simulink model "proyectoscada"  (R2016b)
settings: Solver=VariableStepAuto  StartTime=0.0  StopTime=inf  RelTol=1e-3
undefined symbols (not defined in the file): D1, Delta
libraries: powerlib x32, powerlib_meascontrol x17, sps_avr x2
settings Model: Creator=Chabla  LastModifiedBy=Chabla

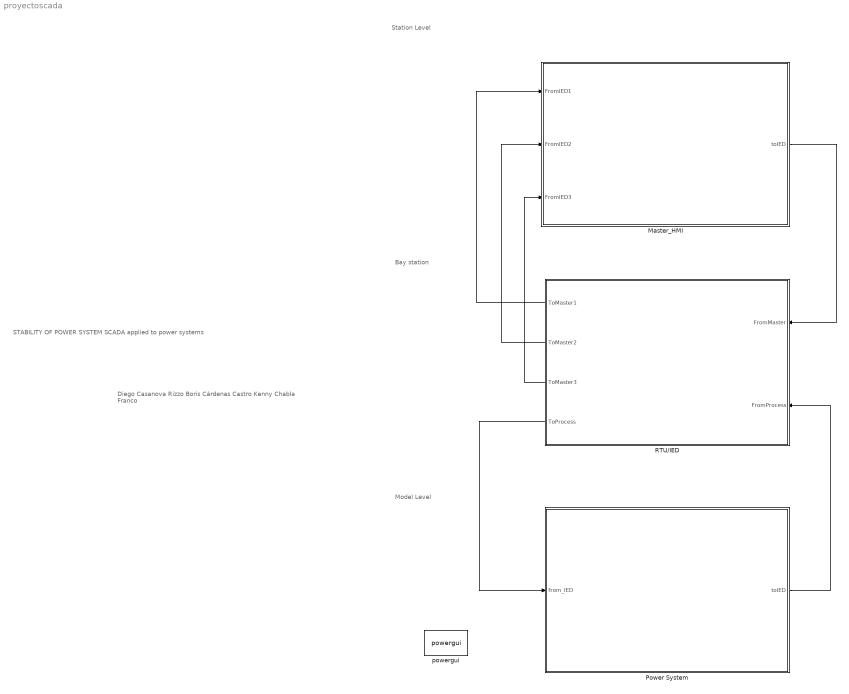
== system proyectoscada ==
  note: Station Level
  note: Bay station
  note: Model Level
  note: STABILITY OF POWER SYSTEM
      | SCADA applied to power systems
  note: Diego Casanova Rizzo
      | Boris Cárdenas Castro
      | Kenny Chabla Franco
  Master_HMI : Subsystem
  Power System : Subsystem
  RTU/IED : Subsystem
  powergui : powerlib/powergui  Priority=1  SimulationMode=Discrete  SolverType=Tustin/Backward Euler (TBE)  SampleTime=50e-6  frequency=60  SPID=off  DisableSnubberDevices=off  DisableRonSwitches=off  DisableVfSwitches=off  SwTol=0  DisplayEquations=off  Interpol=off  ExternalGateDelay=off  methode=off  Ts=10  FunctionMessages=off  echomessages=off  HookPort=off  EnableUseOfTLC=off  x0status=blocks  frequencyindice=60  Pbase=100e6  ErrMax=1e-4  Iterations=50  UnitsV=kV  UnitsW=MW  buscounter=0  RestoreLinks=warning  ResistiveCurrentMeasurement=off  Frange=[0:2:500]  Ylog=off  Xlog=on  ShowGrid=off  save=off  variable=ZData  structure=0  ZoomFFT=off  StartTime=0.0  cycles=1  DisplayStyle=1  fundamental=60  FreqAxis=off  MaxFrequency=1000  frequencyindicesteady=1  RmsSteady=1  display=off
  wires:
  RTU/IED/4(ToProcess) -> Power System/1(from_IED)
  Power System/1(toIED) -> RTU/IED/2(FromProcess)
  RTU/IED/1(ToMaster1) -> Master_HMI/1(FromIED1)
  Master_HMI/1(toIED) -> RTU/IED/1(FromMaster)
  RTU/IED/2(ToMaster2) -> Master_HMI/2(FromIED2)
  RTU/IED/3(ToMaster3) -> Master_HMI/3(FromIED3)

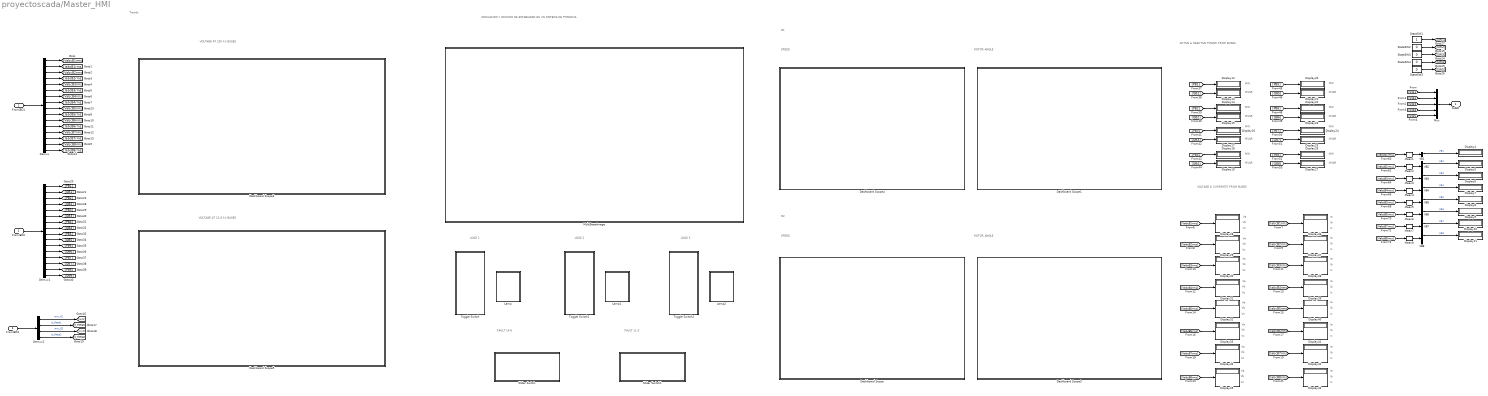
== system proyectoscada/Master_HMI ==
  note: SIMULACIÓN Y ESTUDIO DE ESTABILIDAD
      | EN UN SISTEMA DE POTENCIA
  note: LOAD 1
  note: LOAD 2
  note: LOAD 3
  note: FAULT L4-6
  note: FAULT L1-3
  note: G1
  note: SPEED
  note: ROTOR ANGLE
  note: G2
  note: SPEED
  note: ROTOR ANGLE
  note: ACTIVE & REACTIVE POWER
      | FROM BUSES
  note: VOLTAGE & CURRENTS
      | FROM BUSES
  note: VOLTAGE AT 230 kV BUSES
  note: VOLTAGE AT 13.8 kV BUSES
  note: Trends
  note: MW
  note: MW
  note: MW
  note: MW
  note: MW
  note: MW
  note: MVAR
  note: MVAR
  note: MVAR
  note: MVAR
  note: MVAR
  note: MVAR
  note: MW
  note: MW
  note: MVAR
  note: MVAR
  note: Va
  note: Vb
  note: Vc
  note: Va
  note: Vb
  note: Vc
  note: Va
  note: Vb
  note: Vc
  note: Va
  note: Vb
  note: Vc
  note: Va
  note: Vb
  note: Vc
  note: Va
  note: Vb
  note: Vc
  note: Va
  note: Vb
  note: Vc
  note: Va
  note: Vb
  note: Vc
  note: Ia
  note: Ib
  note: Ic
  note: Ia
  note: Ib
  note: Ic
  note: Ia
  note: Ib
  note: Ic
  note: Ia
  note: Ib
  note: Ic
  note: Ia
  note: Ib
  note: Ic
  note: Ia
  note: Ib
  note: Ic
  note: Ia
  note: Ib
  note: Ic
  note: Ia
  note: Ib
  note: Ic
  FromIED1 : Inport
  FromIED2 : Inport  Port=2
  FromIED3 : Inport  Port=3
  Dashboard Scope : Subsystem  DialogController=hmiCreateDDGDialog  IsWebBlock=on  mask(MWDashboardBlock){webBlockId=cafc33a1-a38a-4801-83e7-bfcad2fb4042, webBlockType=sdiscope, ShowInitialText=on, HMISrcModelName=proyectoscada_primerparcial}
      mask prompts: webBlockId "WebBlock Id"; webBlockType "WebBlock Type"; HMISrcModelName "Source Model"
      mask help: SimulinkHMI:dialogs:HMIScopeDialogDesc
      mask Help: helpview([docroot '/mapfiles/simulink.map'], 'hmi_scope')
      mask Display:
      | if strcmp(get_param(bdroot(gcb),'BlockDiagramType'), 'library')
      |     image([(matlabroot) '/toolbox/simulink/hmi/icons/DashboardScope.png']);
      | end
  Dashboard Scope1 : Subsystem  DialogController=hmiCreateDDGDialog  IsWebBlock=on  mask(MWDashboardBlock){webBlockId=1f27aae5-dc6e-47fc-b79d-12c84d4126a5, webBlockType=sdiscope, ShowInitialText=on, HMISrcModelName=proyectoscada_primerparcial}
      mask prompts: webBlockId "WebBlock Id"; webBlockType "WebBlock Type"; HMISrcModelName "Source Model"
      mask help: SimulinkHMI:dialogs:HMIScopeDialogDesc
      mask Help: helpview([docroot '/mapfiles/simulink.map'], 'hmi_scope')
      mask Display:
      | if strcmp(get_param(bdroot(gcb),'BlockDiagramType'), 'library')
      |     image([(matlabroot) '/toolbox/simulink/hmi/icons/DashboardScope.png']);
      | end
  Dashboard Scope2 : Subsystem  DialogController=hmiCreateDDGDialog  IsWebBlock=on  mask(MWDashboardBlock){webBlockId=bb99fa04-7dbe-4198-be6d-771c31951309, webBlockType=sdiscope, ShowInitialText=off, HMISrcModelName=proyectoscada_primerparcial}
      mask prompts: webBlockId "WebBlock Id"; webBlockType "WebBlock Type"; HMISrcModelName "Source Model"
      mask help: SimulinkHMI:dialogs:HMIScopeDialogDesc
      mask Help: helpview([docroot '/mapfiles/simulink.map'], 'hmi_scope')
      mask Display:
      | if strcmp(get_param(bdroot(gcb),'BlockDiagramType'), 'library')
      |     image([(matlabroot) '/toolbox/simulink/hmi/icons/DashboardScope.png']);
      | end
  Dashboard Scope3 : Subsystem  DialogController=hmiCreateDDGDialog  IsWebBlock=on  mask(MWDashboardBlock){webBlockId=8463cc78-291a-42f6-a448-124f53d8cf61, webBlockType=sdiscope, ShowInitialText=on, HMISrcModelName=proyectoscada_primerparcial}
      mask prompts: webBlockId "WebBlock Id"; webBlockType "WebBlock Type"; HMISrcModelName "Source Model"
      mask help: SimulinkHMI:dialogs:HMIScopeDialogDesc
      mask Help: helpview([docroot '/mapfiles/simulink.map'], 'hmi_scope')
      mask Display:
      | if strcmp(get_param(bdroot(gcb),'BlockDiagramType'), 'library')
      |     image([(matlabroot) '/toolbox/simulink/hmi/icons/DashboardScope.png']);
      | end
  Dashboard Scope4 : Subsystem  DialogController=hmiCreateDDGDialog  IsWebBlock=on  mask(MWDashboardBlock){webBlockId=24e836a3-7620-49fe-a566-1de62ba9f4e1, webBlockType=sdiscope, ShowInitialText=on, HMISrcModelName=proyectoscada_primerparcial}
      mask prompts: webBlockId "WebBlock Id"; webBlockType "WebBlock Type"; HMISrcModelName "Source Model"
      mask help: SimulinkHMI:dialogs:HMIScopeDialogDesc
      mask Help: helpview([docroot '/mapfiles/simulink.map'], 'hmi_scope')
      mask Display:
      | if strcmp(get_param(bdroot(gcb),'BlockDiagramType'), 'library')
      |     image([(matlabroot) '/toolbox/simulink/hmi/icons/DashboardScope.png']);
      | end
  Dashboard Scope5 : Subsystem  DialogController=hmiCreateDDGDialog  IsWebBlock=on  mask(MWDashboardBlock){webBlockId=cad27841-eb8e-42d3-b755-ee1d88cca136, webBlockType=sdiscope, ShowInitialText=off, HMISrcModelName=proyectoscada_primerparcial}
      mask prompts: webBlockId "WebBlock Id"; webBlockType "WebBlock Type"; HMISrcModelName "Source Model"
      mask help: SimulinkHMI:dialogs:HMIScopeDialogDesc
      mask Help: helpview([docroot '/mapfiles/simulink.map'], 'hmi_scope')
      mask Display:
      | if strcmp(get_param(bdroot(gcb),'BlockDiagramType'), 'library')
      |     image([(matlabroot) '/toolbox/simulink/hmi/icons/DashboardScope.png']);
      | end
  Demux : Demux  Outputs=16
  Demux1 : Demux  Outputs=16
  Demux2 : Demux
  Display{4..43} (40 alike) : Display
      settings: Format=bank  Decimation=2
  Lamp : Subsystem  DialogController=hmiCreateDDGDialog  IsWebBlock=on  mask(MWDashboardBlock){webBlockId=6d0128fc-3d43-4d5e-b84a-a99f5afbf392, webBlockType=lamp, ShowInLibBrowser=on, ShowInitialText=on, HMISrcModelName=proyectoscada_primerparcial}
      mask prompts: webBlockType "WebBlock Type"; HMISrcModelName "Source Model"
      mask help: SimulinkHMI:dialogs:LampDialogDesc
      mask Help: helpview([docroot '/mapfiles/simulink.map'], 'hmi_lamp')
      mask Display:
      | if strcmp(get_param(bdroot(gcb),'BlockDiagramType'), 'library')
      |     image([(matlabroot) '/toolbox/simulink/hmi/icons/Lamp.png']);
      | end
  Lamp1 : Subsystem  DialogController=hmiCreateDDGDialog  IsWebBlock=on  mask(MWDashboardBlock){webBlockId=c150fd86-0204-4bcb-8bb8-b9940914ece7, webBlockType=lamp, ShowInLibBrowser=on, ShowInitialText=on, HMISrcModelName=proyectoscada_primerparcial}
      mask prompts: webBlockType "WebBlock Type"; HMISrcModelName "Source Model"
      mask help: SimulinkHMI:dialogs:LampDialogDesc
      mask Help: helpview([docroot '/mapfiles/simulink.map'], 'hmi_lamp')
      mask Display:
      | if strcmp(get_param(bdroot(gcb),'BlockDiagramType'), 'library')
      |     image([(matlabroot) '/toolbox/simulink/hmi/icons/Lamp.png']);
      | end
  Lamp2 : Subsystem  DialogController=hmiCreateDDGDialog  IsWebBlock=on  mask(MWDashboardBlock){webBlockId=436e8146-0c8e-45d0-95ec-43b164432763, webBlockType=lamp, ShowInLibBrowser=on, ShowInitialText=on, HMISrcModelName=proyectoscada_primerparcial}
      mask prompts: webBlockType "WebBlock Type"; HMISrcModelName "Source Model"
      mask help: SimulinkHMI:dialogs:LampDialogDesc
      mask Help: helpview([docroot '/mapfiles/simulink.map'], 'hmi_lamp')
      mask Display:
      | if strcmp(get_param(bdroot(gcb),'BlockDiagramType'), 'library')
      |     image([(matlabroot) '/toolbox/simulink/hmi/icons/Lamp.png']);
      | end
  Mean{1..8} (8 alike) : powerlib_meascontrol/Measurements/Mean  Freq=60  Vinit=0  Ts=0
  MultiStateImage : Subsystem  DialogController=hmiCreateDDGDialog  IsWebBlock=on  mask(MWDashboardBlock){webBlockId=108d4e63-1026-47ee-835d-08ebfdb5bc59, webBlockType=multistateimage, ShowInLibBrowser=on, ShowInitialText=on, HMISrcModelName=proyectoscada_primerparcial}
      mask prompts: webBlockType "WebBlock Type"; HMISrcModelName "Source Model"
      mask help: SimulinkHMI:dialogs:MultiStateImageDialogDesc
      mask Help: helpview([docroot '/mapfiles/simulink.map'], 'hmi_multistateimage')
      mask Display:
      | if strcmp(get_param(bdroot(gcb),'BlockDiagramType'), 'library')
      |     image([(matlabroot) '/toolbox/simulink/hmi/icons/MultiStateImage.png']);
      | end
  Mux : Mux  Inputs=5
  Slider Switch : Subsystem  DialogController=hmiCreateDDGDialog  IsWebBlock=on  mask(MWDashboardBlock){webBlockId=03720d25-6366-4281-ad77-0615db862108, webBlockType=sliderswitch, ShowInLibBrowser=on, ShowInitialText=on, HMISrcModelName=proyectoscada_primerparcial}
      mask prompts: webBlockId "WebBlock Id"; webBlockType "WebBlock Type"; HMISrcModelName "Source Model"
      mask help: SimulinkHMI:dialogs:SwitchDialogDesc
      mask Help: helpview([docroot '/mapfiles/simulink.map'], 'hmi_slider_switch')
      mask Display:
      | if strcmp(get_param(bdroot(gcb),'BlockDiagramType'), 'library')
      |     image([(matlabroot) '/toolbox/simulink/hmi/icons/SliderSwitch.png']);
      | end
  Slider Switch1 : Subsystem  DialogController=hmiCreateDDGDialog  IsWebBlock=on  mask(MWDashboardBlock){webBlockId=6740b061-e7b1-413b-8a03-3a4303ef55f0, webBlockType=sliderswitch, ShowInLibBrowser=on, ShowInitialText=on, HMISrcModelName=proyectoscada_primerparcial}
      mask prompts: webBlockId "WebBlock Id"; webBlockType "WebBlock Type"; HMISrcModelName "Source Model"
      mask help: SimulinkHMI:dialogs:SwitchDialogDesc
      mask Help: helpview([docroot '/mapfiles/simulink.map'], 'hmi_slider_switch')
      mask Display:
      | if strcmp(get_param(bdroot(gcb),'BlockDiagramType'), 'library')
      |     image([(matlabroot) '/toolbox/simulink/hmi/icons/SliderSwitch.png']);
      | end
  StateSW1 : Constant
  StateSW{2..5} (4 alike) : Constant  Value=0
  Toggle Switch : Subsystem  DialogController=hmiCreateDDGDialog  IsWebBlock=on  mask(MWDashboardBlock){webBlockId=0404eeae-805f-465c-bc8a-4052b3d66771, webBlockType=toggleswitch, ShowInLibBrowser=on, ShowInitialText=on, HMISrcModelName=proyectoscada_primerparcial}
      mask prompts: webBlockId "WebBlock Id"; webBlockType "WebBlock Type"; HMISrcModelName "Source Model"
      mask help: SimulinkHMI:dialogs:SwitchDialogDesc
      mask Help: helpview([docroot '/mapfiles/simulink.map'], 'hmi_toggle_switch')
      mask Display:
      | if strcmp(get_param(bdroot(gcb),'BlockDiagramType'), 'library')
      |     image([(matlabroot) '/toolbox/simulink/hmi/icons/ToggleSwitch.png']);
      | end
  Toggle Switch1 : Subsystem  DialogController=hmiCreateDDGDialog  IsWebBlock=on  mask(MWDashboardBlock){webBlockId=4eb36801-e82a-44a6-9453-5649fb68f4bc, webBlockType=toggleswitch, ShowInLibBrowser=on, ShowInitialText=on, HMISrcModelName=proyectoscada_primerparcial}
      mask prompts: webBlockId "WebBlock Id"; webBlockType "WebBlock Type"; HMISrcModelName "Source Model"
      mask help: SimulinkHMI:dialogs:SwitchDialogDesc
      mask Help: helpview([docroot '/mapfiles/simulink.map'], 'hmi_toggle_switch')
      mask Display:
      | if strcmp(get_param(bdroot(gcb),'BlockDiagramType'), 'library')
      |     image([(matlabroot) '/toolbox/simulink/hmi/icons/ToggleSwitch.png']);
      | end
  Toggle Switch2 : Subsystem  DialogController=hmiCreateDDGDialog  IsWebBlock=on  mask(MWDashboardBlock){webBlockId=05c27441-99b6-4173-8686-6e6faba039f7, webBlockType=toggleswitch, ShowInLibBrowser=on, ShowInitialText=on, HMISrcModelName=proyectoscada_primerparcial}
      mask prompts: webBlockId "WebBlock Id"; webBlockType "WebBlock Type"; HMISrcModelName "Source Model"
      mask help: SimulinkHMI:dialogs:SwitchDialogDesc
      mask Help: helpview([docroot '/mapfiles/simulink.map'], 'hmi_toggle_switch')
      mask Display:
      | if strcmp(get_param(bdroot(gcb),'BlockDiagramType'), 'library')
      |     image([(matlabroot) '/toolbox/simulink/hmi/icons/ToggleSwitch.png']);
      | end
  VB{1..8} (8 alike) : Demux  Outputs=3
  toIED : Outport
  wires:
  FromIED1/1 -> Demux/1
  Demux/1 -> [VabcB1rms]
  Demux/2 -> [IabcB1rms]
  Demux/3 -> [VabcB2rms]
  Demux/4 -> [IabcB2rms]
  Demux/5 -> [VabcB3rms]
  Demux/6 -> [IabcB3rms]
  Demux/7 -> [VabcB4rms]
  Demux/8 -> [IabcB4rms]
  Demux/9 -> [VabcB5rms]
  Demux/10 -> [IabcB5rms]
  Demux/11 -> [VabcB6rms]
  Demux/12 -> [IabcB6rms]
  Demux/13 -> [VabcB7rms]
  Demux/14 -> [IabcB7rms]
  Demux/15 -> [VabcB8rms]
  Demux/16 -> [IabcB8rms]
  Demux1/1 -> [PB1]
  Demux1/2 -> [QB1]
  Demux1/3 -> [PB2]
  Demux1/4 -> [QB2]
  Demux1/5 -> [PB3]
  Demux1/6 -> [QB3]
  Demux1/7 -> [PB4]
  Demux1/8 -> [QB4]
  Demux1/9 -> [PB5]
  Demux1/10 -> [QB5]
  Demux1/11 -> [PB6]
  Demux1/12 -> [QB6]
  Demux1/13 -> [PB7]
  Demux1/14 -> [QB7]
  Demux1/15 -> [PB8]
  Demux1/16 -> [QB8]
  FromIED2/1 -> Demux1/1
  Demux2/2 -> [d_theta1]  "d_theta1"
  Demux2/4 -> [d_theta2]  "d_theta2"
  Demux2/1 -> [wm]  "wm_G1"
  Demux2/3 -> [wm2]  "wm_G2"
  FromIED3/1 -> Demux2/1
  Mux/1 -> toIED/1
  [SW1] -> Mux/1
  [SW2] -> Mux/2
  [SW3] -> Mux/3
  [SW4] -> Mux/4
  [SW5] -> Mux/5
  StateSW1/1 -> [SW1]
  StateSW2/1 -> [SW2]
  StateSW3/1 -> [SW3]
  StateSW4/1 -> [SW4]
  StateSW5/1 -> [SW5]
  [VabcB1rms] -> Mean1/1
  Mean1/1 -> VB1/1
  Mean2/1 -> VB2/1
  Mean3/1 -> VB3/1
  Mean4/1 -> VB4/1
  Mean5/1 -> VB5/1
  Mean6/1 -> VB6/1
  Mean7/1 -> VB7/1
  Mean8/1 -> VB8/1
  [VabcB2rms] -> Mean2/1
  [VabcB3rms] -> Mean3/1
  [VabcB4rms] -> Mean4/1
  [VabcB8rms] -> Mean8/1
  [VabcB7rms] -> Mean7/1
  [VabcB6rms] -> Mean6/1
  [VabcB5rms] -> Mean5/1
  VB1/1 -> Display4/1  "VB1"
  VB2/1 -> Display5/1  "VB2"
  VB3/1 -> Display6/1  "VB3"
  VB4/1 -> Display7/1  "VB4"
  VB5/1 -> Display8/1  "VB5"
  VB6/1 -> Display9/1  "VB6"
  VB7/1 -> Display10/1  "VB7"
  VB8/1 -> Display11/1  "VB8"
  [QB1] -> Display13/1
  [PB2] -> Display14/1
  [QB2] -> Display15/1
  [PB3] -> Display16/1
  [QB3] -> Display17/1
  [PB4] -> Display18/1
  [QB4] -> Display19/1
  [PB5] -> Display20/1
  [QB5] -> Display21/1
  [PB6] -> Display22/1
  [QB6] -> Display23/1
  [PB7] -> Display24/1
  [QB7] -> Display25/1
  [PB8] -> Display26/1
  [QB8] -> Display27/1
  [VabcB1rms] -> Display28/1
  [VabcB2rms] -> Display29/1
  [VabcB3rms] -> Display30/1
  [VabcB4rms] -> Display31/1
  [VabcB5rms] -> Display32/1
  [VabcB6rms] -> Display33/1
  [VabcB7rms] -> Display34/1
  [VabcB8rms] -> Display35/1
  [IabcB1rms] -> Display36/1
  [IabcB2rms] -> Display37/1
  [IabcB3rms] -> Display38/1
  [IabcB4rms] -> Display39/1
  [IabcB5rms] -> Display40/1
  [IabcB6rms] -> Display41/1
  [IabcB7rms] -> Display42/1
  [IabcB8rms] -> Display43/1
  [PB1] -> Display12/1

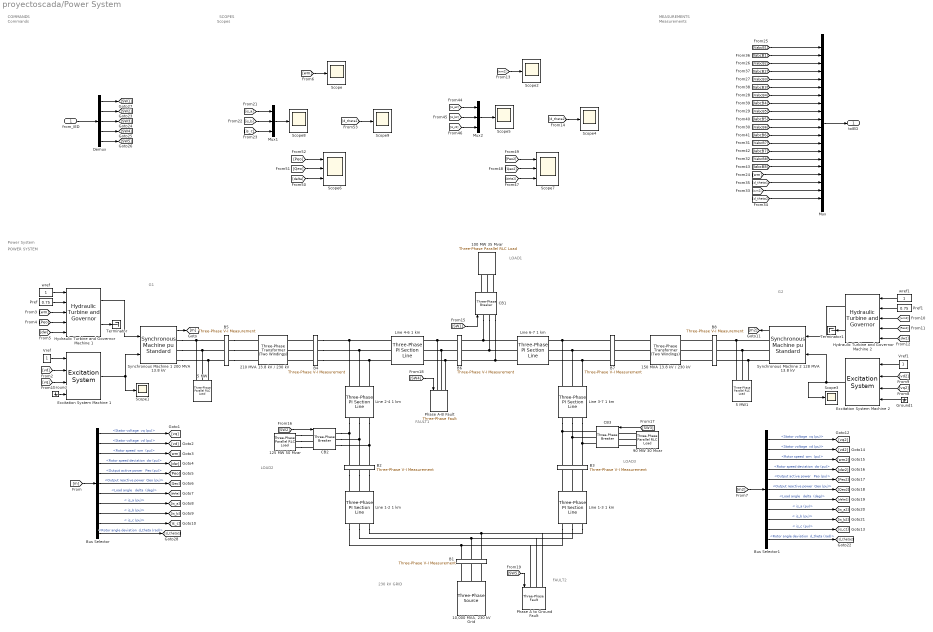
== system proyectoscada/Power System ==
  note: G1
  note: Scopes
  note: Measurements
  note: Power System
  note: Commands
  note: G2
  note: 230 kV
      | GRID
  note: LOAD1
  note: LOAD2
  note: LOAD3
  note: FAULT1
  note: FAULT2
  note: COMMANDS
  note: SCOPES
  note: MEASUREMENTS
  note: POWER SYSTEM
  from_IED : Inport
  "10,000 MVA, 230 kV Grid" : powerlib/Electrical Sources/Three-Phase Source  InternalConnection=Yg  VoltagePhases=off  Voltage=(230000)*1.00006  PhaseAngle=-0.77547  Voltage_phases=[25e3 25e3 25e3]/sqrt(3)  PhaseAngles_phases=[0 -120 +120]  Frequency=60  NonIdealSource=on  SpecifyImpedance=on  Resistance=0.529  Inductance=0.0140  ShortCircuitLevel=10000e6  BaseVoltage=230e3  XRratio=10  BusType=swing  Pref=0  Qref=0  Prefabc=[10e3, 10e3, 10e3]  Qrefabc=[0, 0, 0]  Qmin=-Inf  Qmax=Inf
  100 MW 35 Mvar : powerlib/Elements/Three-Phase Parallel RLC Load  LConnTagsString=A|B|C  Configuration=Y (grounded)  NominalVoltage=230e3  Vabc=[1e3 1e3 1e3]  Vabcp=[1e3 1e3 1e3]  NominalFrequency=60  UnbalancedPower=off  ActivePower=100000000  InductivePower=35000000  CapacitivePower=0  Pabc=[10e3 9e3 11e3]  QLabc=[100 90 110]  QCabc=[100 90 110]  Pabcp=[10e3 9e3 11e3]  QLabcp=[100 90 110]  QCabcp=[100 90 110]  Measurements=None  LoadType=constant Z
  125 MW 50 Mvar : powerlib/Elements/Three-Phase Parallel RLC Load  LConnTagsString=A|B|C  Configuration=Y (grounded)  NominalVoltage=230e3  Vabc=[1e3 1e3 1e3]  Vabcp=[1e3 1e3 1e3]  NominalFrequency=60  UnbalancedPower=off  ActivePower=125000000  InductivePower=50000000  CapacitivePower=0  Pabc=[10e3 9e3 11e3]  QLabc=[100 90 110]  QCabc=[100 90 110]  Pabcp=[10e3 9e3 11e3]  QLabcp=[100 90 110]  QCabcp=[100 90 110]  Measurements=None  LoadType=constant Z
  150 MVA 13.8 kV / 230 kV : powerlib/Elements/Three-Phase Transformer (Two Windings)  Winding1Connection=Delta (D1)  Winding2Connection=Yg  CoreType=Three single-phase transformers  SetSaturation=off  Hysteresis=off  DataFile='hysteresis'  SetInitialFlux=off  Measurements=None  UNITS=pu  NominalPower=[ 150e6 60 ]  Winding1="[ 13.8e3 0.0027  0.08]"  Winding2=[ 230e3 0.0027 0.08]  Rm=500  Lm=500  L0=0.5  Saturation="[ 0,0  ;  0.005,1.2  ;  1.0,1.4 ]"  InitialFluxes=[ 0.8 , -0.8 , 0.7 ]  MoreParameters=off  BreakLoop=off  DataType=off  TransfoNumber=0
  210 MVA 13.8 kV / 230 kV : powerlib/Elements/Three-Phase Transformer (Two Windings)  Winding1Connection=Delta (D1)  Winding2Connection=Yg  CoreType=Three single-phase transformers  SetSaturation=off  Hysteresis=off  DataFile='hysteresis'  SetInitialFlux=off  Measurements=None  UNITS=pu  NominalPower=[ 210e6 60 ]  Winding1="[ 13.8e3 0.0027  0.08]"  Winding2=[ 230e3 0.0027 0.08]  Rm=500  Lm=500  L0=0.5  Saturation="[ 0,0  ;  0.005,1.2  ;  1.0,1.4 ]"  InitialFluxes=[ 0.8 , -0.8 , 0.7 ]  MoreParameters=off  BreakLoop=off  DataType=off  TransfoNumber=0
  5 MW : powerlib/Elements/Three-Phase Parallel RLC Load  LConnTagsString=A|B|C  Configuration=Y (grounded)  NominalVoltage=13.8e3  Vabc=[1e3 1e3 1e3]  Vabcp=[1e3 1e3 1e3]  NominalFrequency=60  UnbalancedPower=off  ActivePower=125000000  InductivePower=0  CapacitivePower=0  Pabc=[10e3 9e3 11e3]  QLabc=[100 90 110]  QCabc=[100 90 110]  Pabcp=[10e3 9e3 11e3]  QLabcp=[100 90 110]  QCabcp=[100 90 110]  Measurements=None  LoadType=constant Z
  5 MW1 : powerlib/Elements/Three-Phase Parallel RLC Load  LConnTagsString=A|B|C  Configuration=Y (grounded)  NominalVoltage=13.8e3  Vabc=[1e3 1e3 1e3]  Vabcp=[1e3 1e3 1e3]  NominalFrequency=60  UnbalancedPower=off  ActivePower=125000000  InductivePower=0  CapacitivePower=0  Pabc=[10e3 9e3 11e3]  QLabc=[100 90 110]  QCabc=[100 90 110]  Pabcp=[10e3 9e3 11e3]  QLabcp=[100 90 110]  QCabcp=[100 90 110]  Measurements=None  LoadType=constant Z
  90 MW 30 Mvar : powerlib/Elements/Three-Phase Parallel RLC Load  LConnTagsString=A|B|C  Configuration=Y (grounded)  NominalVoltage=230e3  Vabc=[1e3 1e3 1e3]  Vabcp=[1e3 1e3 1e3]  NominalFrequency=60  UnbalancedPower=off  ActivePower=90000000  InductivePower=30000000  CapacitivePower=0  Pabc=[10e3 9e3 11e3]  QLabc=[100 90 110]  QCabc=[100 90 110]  Pabcp=[10e3 9e3 11e3]  QLabcp=[100 90 110]  QCabcp=[100 90 110]  Measurements=None  LoadType=constant Z
  B1 : powerlib/Measurements/Three-Phase V-I Measurement  VoltageMeasurement=phase-to-phase  SetLabelV=on  LabelV=VabcB1  Vpu=off  VpuLL=off  CurrentMeasurement=yes  SetLabelI=on  LabelI=IabcB1  Ipu=off  Pbase=100e6  Vbase=500e3  OutputType=Complex  PhasorSimulation=off  PSBequivalent=0
  B2 : powerlib/Measurements/Three-Phase V-I Measurement  VoltageMeasurement=phase-to-phase  SetLabelV=on  LabelV=VabcB2  Vpu=off  VpuLL=off  CurrentMeasurement=yes  SetLabelI=on  LabelI=IabcB2  Ipu=off  Pbase=100e6  Vbase=500e3  OutputType=Complex  PhasorSimulation=off  PSBequivalent=0
  B3 : powerlib/Measurements/Three-Phase V-I Measurement  VoltageMeasurement=phase-to-phase  SetLabelV=on  LabelV=VabcB3  Vpu=off  VpuLL=off  CurrentMeasurement=yes  SetLabelI=on  LabelI=IabcB3  Ipu=off  Pbase=100e6  Vbase=500e3  OutputType=Complex  PhasorSimulation=off  PSBequivalent=0
  B4 : powerlib/Measurements/Three-Phase V-I Measurement  VoltageMeasurement=phase-to-phase  SetLabelV=on  LabelV=VabcB4  Vpu=off  VpuLL=off  CurrentMeasurement=yes  SetLabelI=on  LabelI=IabcB4  Ipu=off  Pbase=100e6  Vbase=500e3  OutputType=Complex  PhasorSimulation=off  PSBequivalent=0
  B5 : powerlib/Measurements/Three-Phase V-I Measurement  VoltageMeasurement=phase-to-phase  SetLabelV=on  LabelV=VabcB5  Vpu=off  VpuLL=off  CurrentMeasurement=yes  SetLabelI=on  LabelI=IabcB5  Ipu=off  Pbase=100e6  Vbase=(13.8e3)  OutputType=Complex  PhasorSimulation=off  PSBequivalent=0
  B6 : powerlib/Measurements/Three-Phase V-I Measurement  VoltageMeasurement=phase-to-phase  SetLabelV=on  LabelV=VabcB6  Vpu=off  VpuLL=off  CurrentMeasurement=yes  SetLabelI=on  LabelI=IabcB6  Ipu=off  Pbase=100e6  Vbase=500e3  OutputType=Complex  PhasorSimulation=off  PSBequivalent=0
  B7 : powerlib/Measurements/Three-Phase V-I Measurement  VoltageMeasurement=phase-to-phase  SetLabelV=on  LabelV=VabcB7  Vpu=off  VpuLL=off  CurrentMeasurement=yes  SetLabelI=on  LabelI=IabcB7  Ipu=off  Pbase=100e6  Vbase=500e3  OutputType=Complex  PhasorSimulation=off  PSBequivalent=0
  B8 : powerlib/Measurements/Three-Phase V-I Measurement  VoltageMeasurement=phase-to-phase  SetLabelV=on  LabelV=VabcB8  Vpu=off  VpuLL=off  CurrentMeasurement=yes  SetLabelI=on  LabelI=IabcB8  Ipu=off  Pbase=100e6  Vbase=500e3  OutputType=Complex  PhasorSimulation=off  PSBequivalent=0
  Bus Selector : BusSelector  OutputSignals="dq0 components.Stator voltage  vq (pu),dq0 components.Stator voltage  vd (pu),Mechanical.Rotor speed  wm  (pu),Mechanical.Rotor speed deviation  dw (pu),Output active power   Peo (pu),Output reactive power  Qeo (pu),Load angle   delta  (deg),Stator current. is_a (pu),Stator current. is_b (pu),Stator current. is_c (pu),Mechanical.Rotor angle deviation  d_theta (rad)"
  Bus Selector1 : BusSelector  OutputSignals="dq0 components.Stator voltage  vq (pu),dq0 components.Stator voltage  vd (pu),Mechanical.Rotor speed  wm  (pu),Mechanical.Rotor speed deviation  dw (pu),Output active power   Peo (pu),Output reactive power  Qeo (pu),Load angle   delta  (deg),Stator current. is_a (pu),Stator current. is_b (pu),Stator current. is_c (pu),Mechanical.Rotor angle deviation  d_theta (rad)"
  CB1 : powerlib/Elements/Three-Phase Breaker  InitialState=closed  SwitchA=on  SwitchB=on  SwitchC=on  SwitchTimes=[14 ]  External=on  BreakerResistance=0.01  SnubberResistance=1e6  SnubberCapacitance=inf  Measurements=None
  CB2 : powerlib/Elements/Three-Phase Breaker  InitialState=closed  SwitchA=on  SwitchB=on  SwitchC=on  SwitchTimes=[14 ]  External=on  BreakerResistance=0.01  SnubberResistance=1e6  SnubberCapacitance=inf  Measurements=None
  CB3 : powerlib/Elements/Three-Phase Breaker  InitialState=closed  SwitchA=on  SwitchB=on  SwitchC=on  SwitchTimes=[14 ]  External=on  BreakerResistance=0.01  SnubberResistance=1e6  SnubberCapacitance=inf  Measurements=None
  Demux : Demux  Outputs=5
  Excitation System Machine 1 : sps_avr/Excitation System  tr=20e-3  reg=[ 300, 0.001 ]  exc=[ 1, 0 ]  tgr=[ 0, 0 ]  damp=[ 0.001, 0.1 ]  sat=[ 0, 0 ]  lim=[ -11.5, 11.5, 0 ]  v0="[1.0  1.28]"
  Excitation System Machine 2 : sps_avr/Excitation System  tr=20e-3  reg=[ 300, 0.001 ]  exc=[ 1, 0 ]  tgr=[ 0, 0 ]  damp=[ 0.001, 0.1 ]  sat=[ 0, 0 ]  lim=[ -11.5, 11.5, 0 ]  v0="[1.0  1.28]"
  Ground : Ground
  Ground1 : Ground
  Hydraulic Turbine and Governor Machine 1 : powerlib/Machines/Hydraulic Turbine and Governor  sm="[ 10/3  0.07 ]"  gate="[  0.01  0.97518  -0.1  0.1 ]"  reg="[  0.05  1.163  0.105  0  0.01  ]"  hyd="[  0  2.67  ]"  dref=0  po=0.7516
  Hydraulic Turbine and Governor Machine 2 : powerlib/Machines/Hydraulic Turbine and Governor  sm="[ 10/3  0.07 ]"  gate="[  0.01  0.97518  -0.1  0.1 ]"  reg="[  0.05  1.163  0.105  0  0.01  ]"  hyd="[  0  2.67  ]"  dref=0  po=0.7516
  Line 1-2 1 km : powerlib/Elements/Three-Phase PI Section Line  LConnTagsString=a|b|c  RConnTagsString=A|B|C  Frequency=60  Resistances=[ 5.29 0]  Inductances="[ 0.119273  0.477092]"  Capacitances=[8.8251416e-7 ((8.8251416e-7)/3)]  Length=1
  Line 1-3 1 km : powerlib/Elements/Three-Phase PI Section Line  LConnTagsString=a|b|c  RConnTagsString=A|B|C  Frequency=60  Resistances=[ 8.993 0]  Inductances="[ 0.129095  0.477092]"  Capacitances=[7.922998e-7 ((7.922998e-7)/3)]  Length=1
  Line 2-4 1 km : powerlib/Elements/Three-Phase PI Section Line  LConnTagsString=a|b|c  RConnTagsString=A|B|C  Frequency=60  Resistances=[ 16.928 0]  Inductances="[ 0.225917  0.477092]"  Capacitances=[1.534386e-6 ((1.534386e-6)/3)]  Length=1
  Line 3-7 1 km : powerlib/Elements/Three-Phase PI Section Line  LConnTagsString=a|b|c  RConnTagsString=A|B|C  Frequency=60  Resistances=[ 20.631 0]  Inductances="[ 0.2385  0.477092]"  Capacitances=[1.7951e-6 ((1.7951e-6)/3)]  Length=1
  Line 4-6 1 km : powerlib/Elements/Three-Phase PI Section Line  LConnTagsString=a|b|c  RConnTagsString=A|B|C  Frequency=60  Resistances=[ 4.4965 0]  Inductances="[ 0.101031  0.477092]"  Capacitances=[7.471263e-7 ((7.471263e-7)/3)]  Length=1
  Line 6-7 1 km : powerlib/Elements/Three-Phase PI Section Line  LConnTagsString=a|b|c  RConnTagsString=A|B|C  Frequency=60  Resistances=[ 6.2951 0]  Inductances="[ 0.141444  0.477092]"  Capacitances=[1.04798e-7 ((1.04798e-7)/3)]  Length=1
  Mux : Mux  Inputs=20
  Mux1 : Mux  Inputs=3
  Mux2 : Mux  Inputs=3
  Phase A to Ground Fault : powerlib/Elements/Three-Phase Fault  InitialStates=0  FaultA=on  FaultB=off  FaultC=off  GroundFault=on  SwitchTimes=[ 7 7.1]  External=on  SwitchStatus=NaN  FaultResistance=1e-3  GroundResistance=1e-3  SnubberResistance=inf  SnubberCapacitance=inf  Measurements=None
  Phase A-B Fault : powerlib/Elements/Three-Phase Fault  InitialStates=0  FaultA=on  FaultB=on  FaultC=off  GroundFault=off  SwitchTimes=[ 7 7.1]  External=on  SwitchStatus=NaN  FaultResistance=1e-3  GroundResistance=1e-3  SnubberResistance=inf  SnubberCapacitance=inf  Measurements=None
  Pref : Constant  Value=0.75
  Pref1 : Constant  Value=0.75
  Scope{,1..5,8..9} (8 alike) : Scope
  Scope6 : Scope  NumInputPorts=3
  Scope7 : Scope  NumInputPorts=3
  Synchronous Machine 1 200 MVA 13.8 kV : powerlib/Machines/Synchronous Machine pu Standard  PresetModel=No  MechanicalLoad=Mechanical power Pm  ShowDetailedParameters=on  RotorType=Salient-pole  Units=per unit standard parameters  MeasurementBus=off  NominalParameters="[ 200E6  13800   60 ]"  Reactances1=[ 31 32 33 34 35 36 37 ]  Reactances2=[ 1.305, 0.296, 0.252, 0.474, 0.243, 0.18 ]  dAxisTimeConstants=Short-circuit  qAxisTimeConstants=Open-circuit  TimeConstants1=[]  TimeConstants2=[]  TimeConstants3=[]  TimeConstants4=[]  TimeConstants5=[ 1.01, 0.053, 0.1 ]  TimeConstants6=[]  TimeConstants7=[]  TimeConstants8=[]  StatorResistance=2.8544e-3  Mechanical=[ 3.2 0 2]  PolePairs=2  InitialConditions=[0 -94.2826 0.750185 0.750185 0.750185 -24.943 -144.943 95.057 1.29071]  SetSaturation=off  Saturation=[0.6404,0.7127,0.8441,0.9214,0.9956,1.082,1.19,1.316,1.457;0.7,0.7698,0.8872,0.9466,0.9969,1.046,1.1,1.151,1.201]  LoadFlowParameters=[1 150000000 0 0]  TsPowergui=0  TsBlock=-1  IterativeModel=Trapezoidal non iterative  IterativeDiscreteModel=Trapezoidal non iterative  BusType=PV  Pref=150000000  Qref=0  Qmin=-Inf  Qmax=Inf  PLF=0  QLF=0
      settings: AttributesFormatString=\n\n
  Synchronous Machine 2 128 MVA 13.8 kV : powerlib/Machines/Synchronous Machine pu Standard  PresetModel=No  MechanicalLoad=Mechanical power Pm  ShowDetailedParameters=on  RotorType=Salient-pole  Units=per unit standard parameters  MeasurementBus=off  NominalParameters="[ 128E6  13800   60 ]"  Reactances1=[ 31 32 33 34 35 36 37 ]  Reactances2=[ 1.68, 0.232064, 0.2, 1.609984, 0.2, 0.094976 ]  dAxisTimeConstants=Short-circuit  qAxisTimeConstants=Open-circuit  TimeConstants1=[]  TimeConstants2=[]  TimeConstants3=[]  TimeConstants4=[]  TimeConstants5=[ 0.81, 0.04, 0.6 ]  TimeConstants6=[]  TimeConstants7=[]  TimeConstants8=[]  StatorResistance=2.8544e-3  Mechanical=[ 3.2 0 2]  PolePairs=2  InitialConditions=[0 -94.2826 0.750185 0.750185 0.750185 -24.943 -144.943 95.057 1.29071]  SetSaturation=off  Saturation=[0.6404,0.7127,0.8441,0.9214,0.9956,1.082,1.19,1.316,1.457;0.7,0.7698,0.8872,0.9466,0.9969,1.046,1.1,1.151,1.201]  LoadFlowParameters=[1 150000000 0 0]  TsPowergui=0  TsBlock=-1  IterativeModel=Trapezoidal non iterative  IterativeDiscreteModel=Trapezoidal non iterative  BusType=PV  Pref=75000000  Qref=0  Qmin=-Inf  Qmax=Inf  PLF=0  QLF=0
      settings: AttributesFormatString=\n\n
  Terminator : Terminator
  Terminator1 : Terminator
  Vref : Constant
  Vref1 : Constant
  wref : Constant
  wref1 : Constant
  toIED : Outport
  wires:
  Demux/4 -> [SW4]
  from_IED/1 -> Demux/1
  Demux/3 -> [SW3]
  Demux/2 -> [SW2]
  Demux/1 -> [SW1]
  [SW3] -> CB3/1
  [SW4] -> Phase A-B Fault/1
  [is_b] -> Mux1/2
  [is_c] -> Mux1/3
  [VabcB1] -> Mux/1
  [VabcB8] -> Mux/15
  [VabcB3] -> Mux/5
  [wm] -> Mux/17
  [VabcB5] -> Mux/9
  [d_theta2] -> Mux/20
  Mux/1 -> toIED/1
  [VabcB2] -> Mux/3
  [VabcB6] -> Mux/11
  [VabcB7] -> Mux/13
  [IabcB5] -> Mux/10
  [IabcB8] -> Mux/16
  [IabcB7] -> Mux/14
  [IabcB6] -> Mux/12
  [delta2] -> Scope7/3
  [Peo2] -> Scope7/1
  [IabcB1] -> Mux/2
  [d_theta1] -> Mux/18
  [IabcB3] -> Mux/6
  [IabcB4] -> Mux/8
  [IabcB2] -> Mux/4
  [d_theta1] -> Scope9/1
  [Peo] -> Scope6/1
  [delta] -> Scope6/3
  [Qeo] -> Scope6/2
  [is_b2] -> Mux2/2
  [is_c2] -> Mux2/3
  [is_a2] -> Mux2/1
  Mux2/1 -> Scope5/1
  [is_a] -> Mux1/1
  Pref/1 -> Hydraulic Turbine and Governor Machine 1/2
  [Qeo2] -> Scope7/2
  Bus Selector/11 -> [d_theta1]  "<Rotor angle deviation  d_theta (rad)>"
  [wm2] -> Mux/19
  [SW2] -> CB2/1
  Excitation System Machine 1/1 -> Scope1/1, Synchronous Machine 1 200 MVA 13.8 kV/2
  Hydraulic Turbine and Governor Machine 1/2 -> Terminator/1
  Hydraulic Turbine and Governor Machine 1/1 -> Synchronous Machine 1 200 MVA 13.8 kV/1
  Vref/1 -> Excitation System Machine 1/1
  [vd] -> Excitation System Machine 1/2
  Bus Selector/6 -> [Qeo]  "<Output reactive power  Qeo (pu)>"
  Bus Selector/7 -> [delta]  "<Load angle   delta  (deg)>"
  Bus Selector/3 -> [wm]  "<Rotor speed  wm  (pu)>"
  Bus Selector/8 -> [is_a]  "< is_a (pu)>"
  Bus Selector/2 -> [vd]  "<Stator voltage  vd (pu)>"
  wref/1 -> Hydraulic Turbine and Governor Machine 1/1
  Bus Selector/4 -> [dw]  "<Rotor speed deviation  dw (pu)>"
  [m] -> Bus Selector/1
  Bus Selector/1 -> [vq]  "<Stator voltage  vq (pu)>"
  Bus Selector/5 -> [Peo]  "<Output active power   Peo (pu)>"
  Synchronous Machine 1 200 MVA 13.8 kV/1 -> [m]
  Ground/1 -> Excitation System Machine 1/4
  Bus Selector/10 -> [is_c]  "< is_c (pu)>"
  Bus Selector/9 -> [is_b]  "< is_b (pu)>"
  [Peo] -> Hydraulic Turbine and Governor Machine 1/4
  [wm] -> Hydraulic Turbine and Governor Machine 1/3
  [wm] -> Scope/1
  [vq] -> Excitation System Machine 1/3
  [dw] -> Hydraulic Turbine and Governor Machine 1/5
  wref1/1 -> Hydraulic Turbine and Governor Machine 2/1
  Pref1/1 -> Hydraulic Turbine and Governor Machine 2/2
  Bus Selector1/6 -> [Qeo2]  "<Output reactive power  Qeo (pu)>"
  [wm2] -> Hydraulic Turbine and Governor Machine 2/3
  Bus Selector1/9 -> [is_b2]  "< is_b (pu)>"
  Bus Selector1/5 -> [Peo2]  "<Output active power   Peo (pu)>"
  Bus Selector1/7 -> [delta2]  "<Load angle   delta  (deg)>"
  Bus Selector1/1 -> [vq2]  "<Stator voltage  vq (pu)>"
  Bus Selector1/3 -> [wm2]  "<Rotor speed  wm  (pu)>"
  Bus Selector1/4 -> [dw2]  "<Rotor speed deviation  dw (pu)>"
  Bus Selector1/8 -> [is_a2]  "< is_a (pu)>"
  [m2] -> Bus Selector1/1
  Bus Selector1/2 -> [vd2]  "<Stator voltage  vd (pu)>"
  Bus Selector1/10 -> [is_c2]  "< is_c (pu)>"
  Hydraulic Turbine and Governor Machine 2/2 -> Terminator1/1
  Ground1/1 -> Excitation System Machine 2/4
  [d_theta2] -> Scope4/1
  [dw2] -> Hydraulic Turbine and Governor Machine 2/5
  Synchronous Machine 2 128 MVA 13.8 kV/1 -> [m2]
  Bus Selector1/11 -> [d_theta2]  "<Rotor angle deviation  d_theta (rad)>"
  [vd2] -> Excitation System Machine 2/2
  Excitation System Machine 2/1 -> Scope3/1, Synchronous Machine 2 128 MVA 13.8 kV/2
  Vref1/1 -> Excitation System Machine 2/1
  Hydraulic Turbine and Governor Machine 2/1 -> Synchronous Machine 2 128 MVA 13.8 kV/1
  [wm2] -> Scope2/1
  [vq2] -> Excitation System Machine 2/3
  [Peo2] -> Hydraulic Turbine and Governor Machine 2/4
  Demux/5 -> [SW5]
  [SW5] -> Phase A to Ground Fault/1
  [SW1] -> CB1/1
  [VabcB4] -> Mux/7
  Mux1/1 -> Scope8/1
  connections:
  90 MW 30 Mvar/LConn3 -- CB3/LConn3
  125 MW 50 Mvar/LConn3 -- CB2/LConn3
  "10,000 MVA, 230 kV Grid"/RConn2 -- B1/LConn2
  B2/LConn2 -- Line 1-2 1 km/RConn2
  Line 1-3 1 km/RConn2 -- B3/LConn2
  B4/RConn3 -- Line 4-6 1 km/LConn3 -- Line 2-4 1 km/RConn3
  "10,000 MVA, 230 kV Grid"/RConn1 -- B1/LConn1
  Line 1-3 1 km/RConn1 -- B3/LConn1
  B2/LConn1 -- Line 1-2 1 km/RConn1
  B4/LConn1 -- 210 MVA 13.8 kV / 230 kV/RConn1
  B5/RConn1 -- 210 MVA 13.8 kV / 230 kV/LConn1
  B4/LConn2 -- 210 MVA 13.8 kV / 230 kV/RConn2
  B2/LConn3 -- Line 1-2 1 km/RConn3
  Line 2-4 1 km/LConn1 -- CB2/RConn1 -- B2/RConn1
  B5/RConn3 -- 210 MVA 13.8 kV / 230 kV/LConn3
  B4/RConn1 -- Line 4-6 1 km/LConn1 -- Line 2-4 1 km/RConn1
  B4/RConn2 -- Line 4-6 1 km/LConn2 -- Line 2-4 1 km/RConn2
  B6/LConn2 -- Phase A-B Fault/LConn2 -- Line 4-6 1 km/RConn2
  "10,000 MVA, 230 kV Grid"/RConn3 -- B1/LConn3
  Line 2-4 1 km/LConn3 -- CB2/RConn3 -- B2/RConn3
  Line 2-4 1 km/LConn2 -- CB2/RConn2 -- B2/RConn2
  B4/LConn3 -- 210 MVA 13.8 kV / 230 kV/RConn3
  Line 1-2 1 km/LConn3 -- Line 1-3 1 km/LConn3 -- Phase A to Ground Fault/LConn3 -- B1/RConn3
  B5/RConn2 -- 210 MVA 13.8 kV / 230 kV/LConn2
  Line 1-2 1 km/LConn1 -- Line 1-3 1 km/LConn1 -- Phase A to Ground Fault/LConn1 -- B1/RConn1
  B6/LConn1 -- Phase A-B Fault/LConn1 -- Line 4-6 1 km/RConn1
  Line 1-3 1 km/RConn3 -- B3/LConn3
  B6/LConn3 -- Phase A-B Fault/LConn3 -- Line 4-6 1 km/RConn3
  Line 1-2 1 km/LConn2 -- Line 1-3 1 km/LConn2 -- Phase A to Ground Fault/LConn2 -- B1/RConn2
  Line 6-7 1 km/LConn2 -- CB1/LConn2 -- B6/RConn2
  Line 6-7 1 km/LConn3 -- CB1/LConn3 -- B6/RConn3
  Synchronous Machine 1 200 MVA 13.8 kV/RConn1 -- 5 MW/LConn1 -- B5/LConn1
  Synchronous Machine 1 200 MVA 13.8 kV/RConn2 -- 5 MW/LConn2 -- B5/LConn2
  Line 3-7 1 km/LConn3 -- CB3/RConn3 -- B3/RConn3
  B7/LConn1 -- Line 3-7 1 km/RConn1 -- Line 6-7 1 km/RConn1
  B7/LConn3 -- Line 3-7 1 km/RConn3 -- Line 6-7 1 km/RConn3
  B8/LConn2 -- 150 MVA 13.8 kV / 230 kV/LConn2
  B8/LConn3 -- 150 MVA 13.8 kV / 230 kV/LConn3
  B8/LConn1 -- 150 MVA 13.8 kV / 230 kV/LConn1
  B7/LConn2 -- Line 3-7 1 km/RConn2 -- Line 6-7 1 km/RConn2
  Line 6-7 1 km/LConn1 -- CB1/LConn1 -- B6/RConn1
  Synchronous Machine 1 200 MVA 13.8 kV/RConn3 -- 5 MW/LConn3 -- B5/LConn3
  Line 3-7 1 km/LConn2 -- CB3/RConn2 -- B3/RConn2
  Line 3-7 1 km/LConn1 -- CB3/RConn1 -- B3/RConn1
  Synchronous Machine 2 128 MVA 13.8 kV/RConn1 -- 5 MW1/LConn1 -- B8/RConn1
  Synchronous Machine 2 128 MVA 13.8 kV/RConn2 -- 5 MW1/LConn2 -- B8/RConn2
  Synchronous Machine 2 128 MVA 13.8 kV/RConn3 -- 5 MW1/LConn3 -- B8/RConn3
  150 MVA 13.8 kV / 230 kV/RConn3 -- B7/RConn3
  CB1/RConn2 -- 100 MW 35 Mvar/LConn2
  CB1/RConn1 -- 100 MW 35 Mvar/LConn1
  150 MVA 13.8 kV / 230 kV/RConn2 -- B7/RConn2
  150 MVA 13.8 kV / 230 kV/RConn1 -- B7/RConn1
  CB1/RConn3 -- 100 MW 35 Mvar/LConn3
  90 MW 30 Mvar/LConn2 -- CB3/LConn2
  125 MW 50 Mvar/LConn2 -- CB2/LConn2
  90 MW 30 Mvar/LConn1 -- CB3/LConn1
  125 MW 50 Mvar/LConn1 -- CB2/LConn1

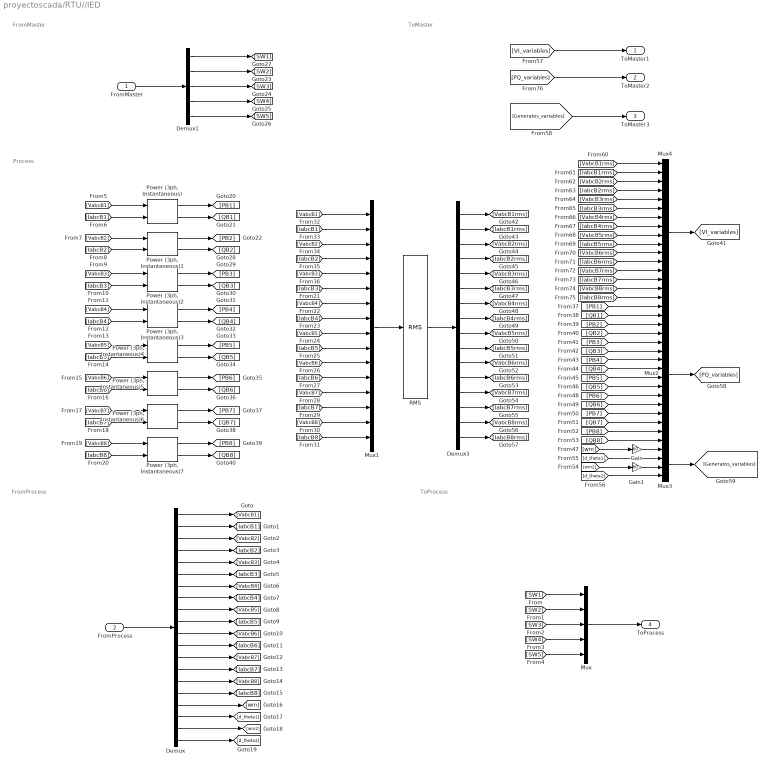
== system proyectoscada/RTU//IED ==
  note: FromMaster
  note: Process
  note: ToMaster
  note: FromProcess
  note: ToProcess
  FromMaster : Inport
  FromProcess : Inport  Port=2
  Demux : Demux  Outputs=20
  Demux1 : Demux  Outputs=5
  Demux3 : Demux  Outputs=16
  Gain : Gain  Gain=60
  Gain1 : Gain  Gain=60
  Mux : Mux  Inputs=5
  Mux1 : Mux  Inputs=16
  Mux2 : Mux  Inputs=16
  Mux3 : Mux
  Mux4 : Mux  Inputs=16
  Power (3ph, Instantaneous){,1..7} (8 alike) : powerlib_meascontrol/Measurements/Power (3ph, Instantaneous)
  RMS : powerlib_meascontrol/Measurements/RMS  TrueRMS=on  Freq=60  RMSInit=120  Ts=0
  ToMaster1 : Outport
  ToMaster2 : Outport  Port=2
  ToMaster3 : Outport  Port=3
  ToProcess : Outport  Port=4
  wires:
  "Power (3ph, Instantaneous)7"/1 -> [PB8]
  [IabcB8] -> "Power (3ph, Instantaneous)7"/2
  [VabcB3] -> Mux1/5
  "Power (3ph, Instantaneous)7"/2 -> [QB8]
  [VabcB8] -> "Power (3ph, Instantaneous)7"/1
  [SW3] -> Mux/3
  [IabcB4] -> Mux1/8
  "Power (3ph, Instantaneous)3"/1 -> [PB4]
  [VabcB4] -> "Power (3ph, Instantaneous)3"/1
  "Power (3ph, Instantaneous)3"/2 -> [QB4]
  [IabcB4] -> "Power (3ph, Instantaneous)3"/2
  [IabcB2] -> Mux1/4
  [SW4] -> Mux/4
  [IabcB3] -> Mux1/6
  [VabcB4] -> Mux1/7
  [IabcB1] -> Mux1/2
  [VabcB1] -> Mux1/1
  Mux4/1 -> [VI_variables]
  [VabcB2] -> Mux1/3
  [VabcB5] -> Mux1/9
  "Power (3ph, Instantaneous)"/2 -> [QB1]
  FromMaster/1 -> Demux1/1
  "Power (3ph, Instantaneous)"/1 -> [PB1]
  [IabcB5] -> "Power (3ph, Instantaneous)4"/2
  [VabcB5] -> "Power (3ph, Instantaneous)4"/1
  "Power (3ph, Instantaneous)4"/1 -> [PB5]
  "Power (3ph, Instantaneous)4"/2 -> [QB5]
  Demux1/4 -> [SW4]
  [VabcB7] -> "Power (3ph, Instantaneous)6"/1
  [IabcB7] -> "Power (3ph, Instantaneous)6"/2
  Demux1/5 -> [SW5]
  Demux1/3 -> [SW3]
  "Power (3ph, Instantaneous)6"/2 -> [QB7]
  "Power (3ph, Instantaneous)6"/1 -> [PB7]
  Demux1/2 -> [SW2]
  Demux1/1 -> [SW1]
  FromProcess/1 -> Demux/1
  [SW5] -> Mux/5
  [SW1] -> Mux/1
  Demux/3 -> [VabcB2]
  Demux/7 -> [VabcB4]
  Demux/18 -> [d_theta1]
  Demux/19 -> [wm2]
  Demux/5 -> [VabcB3]
  Demux/8 -> [IabcB4]
  Demux/9 -> [VabcB5]
  Demux/12 -> [IabcB6]
  Demux/13 -> [VabcB7]
  Demux/1 -> [VabcB1]
  Demux/14 -> [IabcB7]
  Demux/20 -> [d_theta2]
  Demux/2 -> [IabcB1]
  Demux/17 -> [wm]
  Demux/11 -> [VabcB6]
  Demux/4 -> [IabcB2]
  Demux/6 -> [IabcB3]
  Demux/16 -> [IabcB8]
  Demux/15 -> [VabcB8]
  Demux/10 -> [IabcB5]
  Mux/1 -> ToProcess/1
  [VabcB6] -> "Power (3ph, Instantaneous)5"/1
  [SW2] -> Mux/2
  "Power (3ph, Instantaneous)5"/1 -> [PB6]
  "Power (3ph, Instantaneous)5"/2 -> [QB6]
  [IabcB6] -> "Power (3ph, Instantaneous)5"/2
  [IabcB2] -> "Power (3ph, Instantaneous)1"/2
  "Power (3ph, Instantaneous)1"/1 -> [PB2]
  "Power (3ph, Instantaneous)1"/2 -> [QB2]
  [VabcB2] -> "Power (3ph, Instantaneous)1"/1
  [VabcB3] -> "Power (3ph, Instantaneous)2"/1
  "Power (3ph, Instantaneous)2"/1 -> [PB3]
  "Power (3ph, Instantaneous)2"/2 -> [QB3]
  [IabcB3] -> "Power (3ph, Instantaneous)2"/2
  [VI_variables] -> ToMaster1/1
  [IabcB5] -> Mux1/10
  Mux1/1 -> RMS/1
  [VabcB6] -> Mux1/11
  [IabcB8] -> Mux1/16
  [IabcB6] -> Mux1/12
  [IabcB7] -> Mux1/14
  [VabcB7] -> Mux1/13
  [VabcB8] -> Mux1/15
  [VabcB1] -> "Power (3ph, Instantaneous)"/1
  [IabcB1] -> "Power (3ph, Instantaneous)"/2
  RMS/1 -> Demux3/1
  Demux3/1 -> [VabcB1rms]
  Demux3/2 -> [IabcB1rms]
  Demux3/3 -> [VabcB2rms]
  Demux3/4 -> [IabcB2rms]
  Demux3/5 -> [VabcB3rms]
  Demux3/6 -> [IabcB3rms]
  Demux3/7 -> [VabcB4rms]
  Demux3/8 -> [IabcB4rms]
  Demux3/9 -> [VabcB5rms]
  Demux3/10 -> [IabcB5rms]
  Demux3/11 -> [VabcB6rms]
  Demux3/12 -> [IabcB6rms]
  Demux3/13 -> [VabcB7rms]
  Demux3/14 -> [IabcB7rms]
  Demux3/15 -> [VabcB8rms]
  Demux3/16 -> [IabcB8rms]
  [VabcB1rms] -> Mux4/1
  [IabcB1rms] -> Mux4/2
  [VabcB2rms] -> Mux4/3
  [IabcB2rms] -> Mux4/4
  [IabcB4rms] -> Mux4/8
  [VabcB3rms] -> Mux4/5
  [IabcB3rms] -> Mux4/6
  [VabcB4rms] -> Mux4/7
  [VabcB5rms] -> Mux4/9
  [IabcB5rms] -> Mux4/10
  [VabcB6rms] -> Mux4/11
  [IabcB6rms] -> Mux4/12
  [VabcB7rms] -> Mux4/13
  [IabcB7rms] -> Mux4/14
  [VabcB8rms] -> Mux4/15
  [IabcB8rms] -> Mux4/16
  [PB1] -> Mux2/1
  [QB1] -> Mux2/2
  [PB2] -> Mux2/3
  [QB2] -> Mux2/4
  [PB3] -> Mux2/5
  [QB3] -> Mux2/6
  [PB4] -> Mux2/7
  [QB4] -> Mux2/8
  [PB5] -> Mux2/9
  [QB5] -> Mux2/10
  [PB6] -> Mux2/11
  [QB6] -> Mux2/12
  [PB7] -> Mux2/13
  [QB7] -> Mux2/14
  [PB8] -> Mux2/15
  [QB8] -> Mux2/16
  Mux2/1 -> [PQ_variables]
  [PQ_variables] -> ToMaster2/1
  [d_theta1] -> Mux3/2
  [wm] -> Gain/1
  [wm2] -> Gain1/1
  [d_theta2] -> Mux3/4
  Mux3/1 -> [Generatos_variables]
  [Generatos_variables] -> ToMaster3/1
  Gain/1 -> Mux3/1
  Gain1/1 -> Mux3/3

== system proyectoscada/Master_HMI/Dashboard Scope ==

== system proyectoscada/Master_HMI/Dashboard Scope1 ==

== system proyectoscada/Master_HMI/Dashboard Scope2 ==

== system proyectoscada/Master_HMI/Dashboard Scope3 ==

== system proyectoscada/Master_HMI/Dashboard Scope4 ==

== system proyectoscada/Master_HMI/Dashboard Scope5 ==

== system proyectoscada/Master_HMI/Lamp ==

== system proyectoscada/Master_HMI/Lamp1 ==

== system proyectoscada/Master_HMI/Lamp2 ==

== system proyectoscada/Master_HMI/MultiStateImage ==

== system proyectoscada/Master_HMI/Slider Switch ==

== system proyectoscada/Master_HMI/Slider Switch1 ==

== system proyectoscada/Master_HMI/Toggle Switch ==

== system proyectoscada/Master_HMI/Toggle Switch1 ==

== system proyectoscada/Master_HMI/Toggle Switch2 ==
